simulink model "rectifire_single_inverter_pv1"  (R2022b)
settings: Solver=ode23tb  StartTime=0  StopTime=3  RelTol=1e-4
undefined symbols (not defined in the file): Ion, Lithium, P_100, sigbuilder_block, time_step
libraries: spsSeriesRLCBranchLib x26, spsTriangleGeneratorLib x26, slpidlib x26, spsVoltageMeasurementLib x14, spsCurrentMeasurementLib x11, spsDiodeLib x9, simulink x8, spsIGBTDiodeLib x8, spsMosfetLib x8, powerlib_extras x4, spsGroundLib x2, spsBatteryLib x2
(part 5 of 6)

== system rectifire_single_inverter_pv1/battery/Battery and DC-DC converter1/Modulation ==
  u1 : Inport
  u2 : Inport  Port=2
  NOT : Logic  Operator=NOT  AllPortsSameDT=off  OutDataTypeStr=boolean
  NOT1 : Logic  Operator=NOT  AllPortsSameDT=off  OutDataTypeStr=boolean
  Relational Operator : RelationalOperator  Operator=>  OutDataTypeStr=boolean  RndMeth=Simplest  InputSameDT=off
  Relational Operator1 : RelationalOperator  Operator=>  OutDataTypeStr=boolean  RndMeth=Simplest  InputSameDT=off
  Triangle Generator : spsTriangleGeneratorLib/Triangle Generator  Freq=wave_freq  Phase=0  Ts=0
  S1 : Outport
  S2 : Outport  Port=2
  S3 : Outport  Port=3
  S4 : Outport  Port=4
  wires:
  u1/1 -> Relational Operator/1
  Triangle Generator/1 -> Relational Operator1/2, Relational Operator/2
  u2/1 -> Relational Operator1/1
  Relational Operator/1 -> NOT/1, S1/1
  NOT/1 -> S2/1
  Relational Operator1/1 -> S4/1, NOT1/1
  NOT1/1 -> S3/1

== system rectifire_single_inverter_pv1/battery/Battery and DC-DC converter1/Modulation1 ==
  u1 : Inport
  u2 : Inport  Port=2
  NOT : Logic  Operator=NOT  AllPortsSameDT=off  OutDataTypeStr=boolean
  NOT1 : Logic  Operator=NOT  AllPortsSameDT=off  OutDataTypeStr=boolean
  Relational Operator : RelationalOperator  Operator=>  OutDataTypeStr=boolean  RndMeth=Simplest  InputSameDT=off
  Relational Operator1 : RelationalOperator  Operator=>  OutDataTypeStr=boolean  RndMeth=Simplest  InputSameDT=off
  Triangle Generator : spsTriangleGeneratorLib/Triangle Generator  Freq=wave_freq  Phase=0  Ts=0
  S1 : Outport
  S2 : Outport  Port=2
  S3 : Outport  Port=3
  S4 : Outport  Port=4
  wires:
  u1/1 -> Relational Operator/1
  Triangle Generator/1 -> Relational Operator1/2, Relational Operator/2
  u2/1 -> Relational Operator1/1
  Relational Operator/1 -> NOT/1, S1/1
  NOT/1 -> S2/1
  Relational Operator1/1 -> NOT1/1, S3/1
  NOT1/1 -> S4/1

== system rectifire_single_inverter_pv1/battery/Battery and DC-DC converter1/Modulation2 ==
  u1 : Inport
  u2 : Inport  Port=2
  NOT : Logic  Operator=NOT  AllPortsSameDT=off  OutDataTypeStr=boolean
  NOT1 : Logic  Operator=NOT  AllPortsSameDT=off  OutDataTypeStr=boolean
  Relational Operator : RelationalOperator  Operator=>  OutDataTypeStr=boolean  RndMeth=Simplest  InputSameDT=off
  Relational Operator1 : RelationalOperator  Operator=>  OutDataTypeStr=boolean  RndMeth=Simplest  InputSameDT=off
  Triangle Generator : spsTriangleGeneratorLib/Triangle Generator  Freq=wave_freq  Phase=0  Ts=0
  S1 : Outport
  S2 : Outport  Port=2
  S3 : Outport  Port=3
  S4 : Outport  Port=4
  wires:
  u1/1 -> Relational Operator/1
  Triangle Generator/1 -> Relational Operator1/2, Relational Operator/2
  u2/1 -> Relational Operator1/1
  Relational Operator/1 -> NOT/1, S1/1
  NOT/1 -> S2/1
  Relational Operator1/1 -> NOT1/1, S3/1
  NOT1/1 -> S4/1

== system rectifire_single_inverter_pv1/battery/Battery and DC-DC converter1/Modulation3 ==
  u1 : Inport
  u2 : Inport  Port=2
  NOT : Logic  Operator=NOT  AllPortsSameDT=off  OutDataTypeStr=boolean
  NOT1 : Logic  Operator=NOT  AllPortsSameDT=off  OutDataTypeStr=boolean
  Relational Operator : RelationalOperator  Operator=>  OutDataTypeStr=boolean  RndMeth=Simplest  InputSameDT=off
  Relational Operator1 : RelationalOperator  Operator=>  OutDataTypeStr=boolean  RndMeth=Simplest  InputSameDT=off
  Triangle Generator : spsTriangleGeneratorLib/Triangle Generator  Freq=wave_freq  Phase=0  Ts=0
  S1 : Outport
  S2 : Outport  Port=2
  S3 : Outport  Port=3
  S4 : Outport  Port=4
  wires:
  u1/1 -> Relational Operator/1
  Triangle Generator/1 -> Relational Operator1/2, Relational Operator/2
  u2/1 -> Relational Operator1/1
  Relational Operator/1 -> NOT/1, S1/1
  NOT/1 -> S2/1
  Relational Operator1/1 -> NOT1/1, S3/1
  NOT1/1 -> S4/1

== system rectifire_single_inverter_pv1/battery/Battery and DC-DC converter1/Modulation4 ==
  u1 : Inport
  u2 : Inport  Port=2
  NOT : Logic  Operator=NOT  AllPortsSameDT=off  OutDataTypeStr=boolean
  NOT1 : Logic  Operator=NOT  AllPortsSameDT=off  OutDataTypeStr=boolean
  Relational Operator : RelationalOperator  Operator=>  OutDataTypeStr=boolean  RndMeth=Simplest  InputSameDT=off
  Relational Operator1 : RelationalOperator  Operator=>  OutDataTypeStr=boolean  RndMeth=Simplest  InputSameDT=off
  Triangle Generator : spsTriangleGeneratorLib/Triangle Generator  Freq=wave_freq  Phase=0  Ts=0
  S1 : Outport
  S2 : Outport  Port=2
  S3 : Outport  Port=3
  S4 : Outport  Port=4
  wires:
  u1/1 -> Relational Operator/1
  Triangle Generator/1 -> Relational Operator1/2, Relational Operator/2
  u2/1 -> Relational Operator1/1
  Relational Operator/1 -> NOT/1, S1/1
  NOT/1 -> S2/1
  Relational Operator1/1 -> NOT1/1, S3/1
  NOT1/1 -> S4/1

== system rectifire_single_inverter_pv1/battery/Battery and DC-DC converter1/Modulation5 ==
  u1 : Inport
  u2 : Inport  Port=2
  NOT : Logic  Operator=NOT  AllPortsSameDT=off  OutDataTypeStr=boolean
  NOT1 : Logic  Operator=NOT  AllPortsSameDT=off  OutDataTypeStr=boolean
  Relational Operator : RelationalOperator  Operator=>  OutDataTypeStr=boolean  RndMeth=Simplest  InputSameDT=off
  Relational Operator1 : RelationalOperator  Operator=>  OutDataTypeStr=boolean  RndMeth=Simplest  InputSameDT=off
  Triangle Generator : spsTriangleGeneratorLib/Triangle Generator  Freq=wave_freq  Phase=0  Ts=0
  S1 : Outport
  S2 : Outport  Port=2
  S3 : Outport  Port=3
  S4 : Outport  Port=4
  wires:
  u1/1 -> Relational Operator/1
  Triangle Generator/1 -> Relational Operator1/2, Relational Operator/2
  u2/1 -> Relational Operator1/1
  Relational Operator/1 -> NOT/1, S1/1
  NOT/1 -> S2/1
  Relational Operator1/1 -> NOT1/1, S3/1
  NOT1/1 -> S4/1

== system rectifire_single_inverter_pv1/battery/Battery and DC-DC converter1/Modulation6 ==
  u1 : Inport
  u2 : Inport  Port=2
  NOT : Logic  Operator=NOT  AllPortsSameDT=off  OutDataTypeStr=boolean
  NOT1 : Logic  Operator=NOT  AllPortsSameDT=off  OutDataTypeStr=boolean
  Relational Operator : RelationalOperator  Operator=>  OutDataTypeStr=boolean  RndMeth=Simplest  InputSameDT=off
  Relational Operator1 : RelationalOperator  Operator=>  OutDataTypeStr=boolean  RndMeth=Simplest  InputSameDT=off
  Triangle Generator : spsTriangleGeneratorLib/Triangle Generator  Freq=wave_freq  Phase=0  Ts=0
  S1 : Outport
  S2 : Outport  Port=2
  S3 : Outport  Port=3
  S4 : Outport  Port=4
  wires:
  u1/1 -> Relational Operator/1
  Triangle Generator/1 -> Relational Operator1/2, Relational Operator/2
  u2/1 -> Relational Operator1/1
  Relational Operator/1 -> NOT/1, S1/1
  NOT/1 -> S2/1
  Relational Operator1/1 -> NOT1/1, S3/1
  NOT1/1 -> S4/1

== system rectifire_single_inverter_pv1/inverter/Subsystem/PWM1 ==
  In1 : Inport
  In2 : Inport  Port=2
  Constant : Constant
  Constant1 : Constant  Value=0
  Data Type Conversion1 : DataTypeConversion  OutDataTypeStr=boolean
  Subtract : Sum  Inputs=+-
  Switch : Switch  Threshold=0.5  SaturateOnIntegerOverflow=off  InputSameDT=off
  Out1 : Outport
  wires:
  Constant/1 -> Switch/1
  Subtract/1 -> Switch/2
  In2/1 -> Subtract/2
  In1/1 -> Subtract/1
  Switch/1 -> Data Type Conversion1/1
  Data Type Conversion1/1 -> Out1/1
  Constant1/1 -> Switch/3

== system rectifire_single_inverter_pv1/motor/SVPWM/PWM ==
  In : Inport
  Tcm123 : Inport  Port=2
  Add : Sum  Inputs=+-
  Add1 : Sum  Inputs=+-
  Add2 : Sum  Inputs=+-
  Data Type Conversion : DataTypeConversion  OutDataTypeStr=double  SaturateOnIntegerOverflow=off  RndMeth=Floor
  Data Type Conversion1 : DataTypeConversion  OutDataTypeStr=double  SaturateOnIntegerOverflow=off  RndMeth=Floor
  Data Type Conversion2 : DataTypeConversion  OutDataTypeStr=double  SaturateOnIntegerOverflow=off  RndMeth=Floor
  Demux : Demux  Outputs=3
  Logical Operator : Logic  Operator=NOT  AllPortsSameDT=off  OutDataTypeStr=boolean
  Logical Operator1 : Logic  Operator=NOT  AllPortsSameDT=off  OutDataTypeStr=boolean
  Logical Operator2 : Logic  Operator=NOT  AllPortsSameDT=off  OutDataTypeStr=boolean
  Mux : Mux  Inputs=6
  Relay : Relay  OffSwitchValue=-eps
  Relay1 : Relay  OffSwitchValue=-eps
  Relay2 : Relay  OffSwitchValue=-eps
  PWM : Outport  VectorParamsAs1DForOutWhenUnconnected=off
  wires:
  Demux/3 -> Add2/2
  Demux/2 -> Add1/2
  Demux/1 -> Add/2
  Relay2/1 -> Mux/5, Logical Operator2/1
  Relay1/1 -> Mux/3, Logical Operator1/1
  Relay/1 -> Logical Operator/1, Mux/1
  Mux/1 -> PWM/1
  Data Type Conversion/1 -> Mux/2
  Data Type Conversion1/1 -> Mux/4
  Data Type Conversion2/1 -> Mux/6
  Logical Operator2/1 -> Data Type Conversion2/1
  Logical Operator1/1 -> Data Type Conversion1/1
  Logical Operator/1 -> Data Type Conversion/1
  Add1/1 -> Relay1/1
  Add2/1 -> Relay2/1
  Add/1 -> Relay/1
  In/1 -> Add/1, Add2/1, Add1/1
  Tcm123/1 -> Demux/1

== system rectifire_single_inverter_pv1/motor/SVPWM/Sector Caculate ==
  Ualpha : Inport
  Ubeta : Inport  Port=2
  B0 : Fcn  Expr=u[2]
  B1 : Fcn  Expr=u[1]*sqrt(3/4)-0.5*u[2]
  B2 : Fcn  Expr=-u[1]*sqrt(3/4)-u[2]*0.5
  Constant : Constant
  Constant1 : Constant  Value=0
  Mux : Mux  Inputs=2
  Mux1 : Mux  Inputs=3
  N : Fcn  Expr=4*u[3]+2*u[2]+u[1]
  Switch : Switch  SaturateOnIntegerOverflow=off  InputSameDT=off
  Switch1 : Switch  SaturateOnIntegerOverflow=off  InputSameDT=off
  Switch2 : Switch  SaturateOnIntegerOverflow=off  InputSameDT=off
  "N " : Outport  VectorParamsAs1DForOutWhenUnconnected=off
  wires:
  Switch2/1 -> Mux1/3
  Switch/1 -> Mux1/1
  Ualpha/1 -> Mux/1
  Ubeta/1 -> Mux/2
  Mux/1 -> B2/1, B1/1, B0/1
  B0/1 -> Switch/2
  B1/1 -> Switch1/2
  B2/1 -> Switch2/2
  Constant/1 -> Switch/1, Switch2/1, Switch1/1
  Constant1/1 -> Switch/3, Switch1/3, Switch2/3
  Switch1/1 -> Mux1/2
  Mux1/1 -> N/1
  N/1 -> "N "/1

== system rectifire_single_inverter_pv1/motor/SVPWM/T1T1 Caculate ==
  note: T1
  note: T2
  N : Inport
  XYZ : Inport  Port=2
  Tpwm : Inport  Port=3
  Demux : Demux  Outputs=3
  Fcn : Fcn  Expr=u(3)-u(2)-u(1)
  Fcn1 : Fcn  Expr=u(1)*u(3)/(u(1)+u(2))
  Fcn2 : Fcn  Expr=u(2)*u(3)/(u(1)+u(2))
  Gain : Gain  Gain=-1
  Gain1 : Gain  Gain=-1
  Gain2 : Gain  Gain=-1
  Multiport Switch : MultiPortSwitch  Inputs=6  DiagnosticForDefault=None  SaturateOnIntegerOverflow=off  InputSameDT=off
  Multiport Switch1 : MultiPortSwitch  Inputs=6  DiagnosticForDefault=None  SaturateOnIntegerOverflow=off  InputSameDT=off
  Mux : Mux  Inputs=3
  Switch : Switch  SaturateOnIntegerOverflow=off  InputSameDT=off
  Switch1 : Switch  Criteria=u2 > Threshold  SaturateOnIntegerOverflow=off  InputSameDT=off
  T1 : Outport  VectorParamsAs1DForOutWhenUnconnected=off
  T2 : Outport  Port=2  VectorParamsAs1DForOutWhenUnconnected=off
  wires:
  Tpwm/1 -> Mux/3
  XYZ/1 -> Demux/1
  Switch1/1 -> T2/1
  Switch/1 -> T1/1
  Fcn2/1 -> Switch1/3
  Fcn1/1 -> Switch/3
  Fcn/1 -> Switch/2, Switch1/2
  Mux/1 -> Fcn1/1, Fcn/1, Fcn2/1
  Multiport Switch/1 -> Switch/1, Mux/1
  Multiport Switch1/1 -> Switch1/1, Mux/2
  N/1 -> Multiport Switch/1, Multiport Switch1/1
  Demux/2 -> Multiport Switch/3, Multiport Switch1/2, Gain1/1
  Demux/3 -> Multiport Switch1/5, Multiport Switch/2, Gain2/1
  Demux/1 -> Multiport Switch/6, Multiport Switch1/4, Gain/1
  Gain/1 -> Multiport Switch1/3, Multiport Switch/5
  Gain2/1 -> Multiport Switch/4, Multiport Switch1/7
  Gain1/1 -> Multiport Switch1/6, Multiport Switch/7

== system rectifire_single_inverter_pv1/motor/SVPWM/Tcm Caculate ==
  N : Inport
  T1 : Inport  Port=2
  T2 : Inport  Port=3
  Tpwm : Inport  Port=4
  Fcn : Fcn  Expr=(u[3]-u[1]-u[2])/4
  Fcn1 : Fcn  Expr=(u[3]+u[1]-u[2])/4
  Fcn2 : Fcn  Expr=(u[3]+u[2]+u[1])/4
  Multiport Switch : MultiPortSwitch  Inputs=6  DiagnosticForDefault=None  SaturateOnIntegerOverflow=off  InputSameDT=off
  Multiport Switch1 : MultiPortSwitch  Inputs=6  DiagnosticForDefault=None  SaturateOnIntegerOverflow=off  InputSameDT=off
  Multiport Switch2 : MultiPortSwitch  Inputs=6  DiagnosticForDefault=None  SaturateOnIntegerOverflow=off  InputSameDT=off
  Mux : Mux  Inputs=3
  Mux1 : Mux  Inputs=3
  Tcm1 Tcm2 Tcm3 : Outport  VectorParamsAs1DForOutWhenUnconnected=off
  wires:
  Mux/1 -> Fcn2/1, Fcn/1, Fcn1/1
  Tpwm/1 -> Mux/3
  T2/1 -> Mux/2
  T1/1 -> Mux/1
  Multiport Switch2/1 -> Mux1/3
  Multiport Switch1/1 -> Mux1/2
  Multiport Switch/1 -> Mux1/1
  Mux1/1 -> Tcm1 Tcm2 Tcm3/1
  Fcn/1 -> Multiport Switch/3, Multiport Switch/4, Multiport Switch1/6, Multiport Switch2/5, Multiport Switch2/7, Multiport Switch1/2
  Fcn1/1 -> Multiport Switch1/5, Multiport Switch2/3, Multiport Switch2/6, Multiport Switch1/4, Multiport Switch/7, Multiport Switch/2
  Fcn2/1 -> Multiport Switch/5, Multiport Switch/6, Multiport Switch1/3, Multiport Switch1/7, Multiport Switch2/2, Multiport Switch2/4
  N/1 -> Multiport Switch2/1, Multiport Switch1/1, Multiport Switch/1

== system rectifire_single_inverter_pv1/motor/SVPWM/XYZ Caculate ==
  Ualpha : Inport
  Ubeta : Inport  Port=2
  Ts : Inport  Port=3
  Udc : Inport  Port=4
  Add : Sum
  Add1 : Sum  Inputs=+-
  Gain : Gain  Gain=3/2
  Gain1 : Gain  Gain=sqrt(3)
  Gain2 : Gain  Gain=sqrt(3)/2
  Math Function : Math  Operator=reciprocal  SignedPower=on
  Mux : Mux  Inputs=3
  Product{,1..3} (4 alike) : Product  RndMeth=Zero
  XYZ : Outport  VectorParamsAs1DForOutWhenUnconnected=off
  wires:
  Mux/1 -> XYZ/1
  Product1/1 -> Mux/1
  Product3/1 -> Mux/2
  Product2/1 -> Mux/3
  Ualpha/1 -> Gain/1
  Ubeta/1 -> Gain2/1, Gain1/1
  Udc/1 -> Math Function/1
  Math Function/1 -> Product/2
  Ts/1 -> Product/1
  Gain1/1 -> Product1/1
  Product/1 -> Product2/2, Product1/2, Product3/2
  Gain/1 -> Add1/2, Add/2
  Gain2/1 -> Add/1, Add1/1
  Add1/1 -> Product2/1
  Add/1 -> Product3/1

== system rectifire_single_inverter_pv1/PV/PV module/PV module1/PV Current ==
  V : Inport
  T : Inport  Port=2
  I0 : Inport  Port=3
  Iph : Inport  Port=4
  Ish : Inport  Port=5
  Add1 : Sum
  Add2 : Sum  Inputs=+-
  Add3 : Sum  Inputs=+--
  Constant1 : Constant  Value=Rs
  Constant2 : Constant  Value=q
  Constant3 : Constant  Value=n
  Constant4 : Constant  Value=K
  Constant5 : Constant  Value=Ns
  Constant6 : Constant
  Math Function1 : Math
  Memory : Memory
  Product1 : Product
  Product2 : Product  Inputs=*////
  Product3 : Product
  Product4 : Product
  I : Outport
  wires:
  Add1/1 -> Product3/1
  V/1 -> Add1/1
  Add3/1 -> Memory/1, I/1
  Add2/1 -> Product4/2
  Product3/1 -> Math Function1/1
  Iph/1 -> Add3/1
  Product1/1 -> Add1/2
  Constant1/1 -> Product1/2
  Math Function1/1 -> Add2/1
  T/1 -> Product2/5
  Product2/1 -> Product3/2
  Constant5/1 -> Product2/4
  Constant3/1 -> Product2/2
  Constant4/1 -> Product2/3
  Constant2/1 -> Product2/1
  Product4/1 -> Add3/2
  I0/1 -> Product4/1
  Constant6/1 -> Add2/2
  Ish/1 -> Add3/3
  Memory/1 -> Product1/1

== system rectifire_single_inverter_pv1/PV/PV module/PV module1/Photo-current ==
  T : Inport
  G : Inport  Port=2
  Add1 : Sum  Inputs=+-
  Add2 : Sum
  Constant1 : Constant  Value=298
  Constant2 : Constant  Value=ki
  Constant3 : Constant  Value=Isc
  Constant4 : Constant  Value=1000
  Product1 : Product
  Product2 : Product
  Product3 : Product  Inputs=*/
  Iph : Outport
  wires:
  T/1 -> Add1/1
  G/1 -> Product2/1
  Product1/1 -> Add2/2
  Constant4/1 -> Product3/2
  Constant2/1 -> Product1/2
  Product3/1 -> Iph/1
  Constant3/1 -> Add2/1
  Add1/1 -> Product1/1
  Constant1/1 -> Add1/2
  Add2/1 -> Product2/2
  Product2/1 -> Product3/1

== system rectifire_single_inverter_pv1/PV/PV module/PV module1/Reverse Saturation Current ==
  T : Inport
  Add : Sum  Inputs=+-
  Constant2 : Constant  Value=q  SampleTime=-1
  Constant3 : Constant  Value=Voc  SampleTime=-1
  Constant4 : Constant  Value=n  SampleTime=-1
  Constant5 : Constant  VectorParams1D=off  SampleTime=-1
  Constant6 : Constant  Value=K  SampleTime=-1
  Constant7 : Constant  Value=Ns  SampleTime=-1
  Constant8 : Constant  Value=Isc  SampleTime=-1
  Math Function1 : Math
  Product1 : Product
  Product2 : Product  Inputs=4
  Product3 : Product  Inputs=*/
  Product4 : Product  Inputs=*/
  Irc : Outport
  wires:
  Product4/1 -> Irc/1
  Product2/1 -> Product3/2
  T/1 -> Product2/4
  Constant5/1 -> Add/2
  Constant2/1 -> Product1/1
  Product3/1 -> Math Function1/1
  Add/1 -> Product4/2
  Constant8/1 -> Product4/1
  Constant3/1 -> Product1/2
  Constant7/1 -> Product2/2
  Constant4/1 -> Product2/1
  Constant6/1 -> Product2/3
  Math Function1/1 -> Add/1
  Product1/1 -> Product3/1

== system rectifire_single_inverter_pv1/PV/PV module/PV module1/Saturation current ==
  T : Inport
  Irs : Inport  Port=2
  Add : Sum  Inputs=+-
  Constant10 : Constant  Value=3  VectorParams1D=off  SampleTime=-1
  Constant2 : Constant  VectorParams1D=off  SampleTime=-1
  Constant3 : Constant  Value=Tn  SampleTime=-1
  Constant4 : Constant  VectorParams1D=off  SampleTime=-1
  Constant5 : Constant  Value=q  SampleTime=-1
  Constant6 : Constant  Value=Eg0  SampleTime=-1
  Constant7 : Constant  Value=n  SampleTime=-1
  Constant8 : Constant  Value=K  SampleTime=-1
  Constant9 : Constant  Value=Tn  SampleTime=-1
  Math Function1 : Math
  Math Function2 : Math  Operator=pow
  Product{1..2,5..6} (4 alike) : Product  Inputs=*/
  Product3 : Product  Inputs=3
  Product4 : Product
  Product7 : Product  Inputs=3
  I0 : Outport
  wires:
  T/1 -> Product2/2, Product6/1
  Constant7/1 -> Product4/1
  Product6/1 -> Math Function2/1
  Math Function1/1 -> Product7/3
  Constant2/1 -> Product1/1
  Constant4/1 -> Product2/1
  Product3/1 -> Product5/1
  Add/1 -> Product3/3
  Irs/1 -> Product7/1
  Constant3/1 -> Product1/2
  Math Function2/1 -> Product7/2
  Constant10/1 -> Math Function2/2
  Product1/1 -> Add/1
  Constant8/1 -> Product4/2
  Constant9/1 -> Product6/2
  Product4/1 -> Product5/2
  Constant6/1 -> Product3/2
  Product7/1 -> I0/1
  Product5/1 -> Math Function1/1
  Constant5/1 -> Product3/1
  Product2/1 -> Add/2

== system rectifire_single_inverter_pv1/PV/PV module/PV module1/Shunt Current ==
  I : Inport
  V : Inport  Port=2
  Add : Sum
  Constant1 : Constant  Value=Rs  SampleTime=-1
  Constant2 : Constant  Value=Rsh  SampleTime=-1
  Product1 : Product
  Product2 : Product  Inputs=*/
  Ish : Outport
  wires:
  I/1 -> Product1/1
  Constant1/1 -> Product1/2
  Product2/1 -> Ish/1
  Constant2/1 -> Product2/2
  V/1 -> Add/2
  Add/1 -> Product2/1
  Product1/1 -> Add/1

== system rectifire_single_inverter_pv1/battery/Battery and DC-DC converter/Charge Mixed CurrentPower/Modulation ==
  u1 : Inport
  u2 : Inport  Port=2
  triangular_generator : Inport  Port=3
  NOT : Logic  Operator=NOT  AllPortsSameDT=off  OutDataTypeStr=boolean
  NOT1 : Logic  Operator=NOT  AllPortsSameDT=off  OutDataTypeStr=boolean
  Relational Operator : RelationalOperator  Operator=>  OutDataTypeStr=boolean  RndMeth=Simplest  InputSameDT=off
  Relational Operator1 : RelationalOperator  Operator=>  OutDataTypeStr=boolean  RndMeth=Simplest  InputSameDT=off
  Triangle Generator : spsTriangleGeneratorLib/Triangle Generator  Commented=on  Freq=wave_freq  Phase=0  Ts=0
  S1 : Outport
  S2 : Outport  Port=2
  S3 : Outport  Port=3
  S4 : Outport  Port=4
  wires:
  u1/1 -> Relational Operator/1
  triangular_generator/1 -> Relational Operator1/2, Relational Operator/2
  u2/1 -> Relational Operator1/1
  NOT1/1 -> S4/1
  Relational Operator/1 -> S1/1, NOT/1
  Relational Operator1/1 -> S3/1, NOT1/1
  NOT/1 -> S2/1

== system rectifire_single_inverter_pv1/battery/Battery and DC-DC converter/Charge Mixed CurrentPower1/Modulation ==
  u1 : Inport
  u2 : Inport  Port=2
  triangular_generator : Inport  Port=3
  NOT : Logic  Operator=NOT  AllPortsSameDT=off  OutDataTypeStr=boolean
  NOT1 : Logic  Operator=NOT  AllPortsSameDT=off  OutDataTypeStr=boolean
  Relational Operator : RelationalOperator  Operator=>  OutDataTypeStr=boolean  RndMeth=Simplest  InputSameDT=off
  Relational Operator1 : RelationalOperator  Operator=>  OutDataTypeStr=boolean  RndMeth=Simplest  InputSameDT=off
  Triangle Generator : spsTriangleGeneratorLib/Triangle Generator  Commented=on  Freq=wave_freq  Phase=0  Ts=0
  S1 : Outport
  S2 : Outport  Port=2
  S3 : Outport  Port=3
  S4 : Outport  Port=4
  wires:
  u1/1 -> Relational Operator/1
  triangular_generator/1 -> Relational Operator1/2, Relational Operator/2
  u2/1 -> Relational Operator1/1
  NOT1/1 -> S4/1
  Relational Operator/1 -> S1/1, NOT/1
  Relational Operator1/1 -> S3/1, NOT1/1
  NOT/1 -> S2/1

== system rectifire_single_inverter_pv1/battery/Battery and DC-DC converter/Discharge Const Voltage/Modulation ==
  u1 : Inport
  u2 : Inport  Port=2
  triangular_generator : Inport  Port=3
  NOT : Logic  Operator=NOT  AllPortsSameDT=off  OutDataTypeStr=boolean
  NOT1 : Logic  Operator=NOT  AllPortsSameDT=off  OutDataTypeStr=boolean
  Relational Operator : RelationalOperator  Operator=>  OutDataTypeStr=boolean  RndMeth=Simplest  InputSameDT=off
  Relational Operator1 : RelationalOperator  Operator=>  OutDataTypeStr=boolean  RndMeth=Simplest  InputSameDT=off
  Triangle Generator : spsTriangleGeneratorLib/Triangle Generator  Commented=on  Freq=wave_freq  Phase=0  Ts=0
  S1 : Outport
  S2 : Outport  Port=2
  S3 : Outport  Port=3
  S4 : Outport  Port=4
  wires:
  u1/1 -> Relational Operator/1
  triangular_generator/1 -> Relational Operator1/2, Relational Operator/2
  u2/1 -> Relational Operator1/1
  NOT1/1 -> S4/1
  Relational Operator/1 -> S1/1, NOT/1
  Relational Operator1/1 -> S3/1, NOT1/1
  NOT/1 -> S2/1

== system rectifire_single_inverter_pv1/battery/Battery and DC-DC converter/Discharge Mixed CurrentPower/Modulation ==
  u1 : Inport
  u2 : Inport  Port=2
  triangular_generator : Inport  Port=3
  NOT : Logic  Operator=NOT  AllPortsSameDT=off  OutDataTypeStr=boolean
  NOT1 : Logic  Operator=NOT  AllPortsSameDT=off  OutDataTypeStr=boolean
  Relational Operator : RelationalOperator  Operator=>  OutDataTypeStr=boolean  RndMeth=Simplest  InputSameDT=off
  Relational Operator1 : RelationalOperator  Operator=>  OutDataTypeStr=boolean  RndMeth=Simplest  InputSameDT=off
  Triangle Generator : spsTriangleGeneratorLib/Triangle Generator  Commented=on  Freq=wave_freq  Phase=0  Ts=0
  S1 : Outport
  S2 : Outport  Port=2
  S3 : Outport  Port=3
  S4 : Outport  Port=4
  wires:
  u1/1 -> Relational Operator/1
  triangular_generator/1 -> Relational Operator1/2, Relational Operator/2
  u2/1 -> Relational Operator1/1
  NOT1/1 -> S4/1
  Relational Operator/1 -> S1/1, NOT/1
  Relational Operator1/1 -> S3/1, NOT1/1
  NOT/1 -> S2/1

== system rectifire_single_inverter_pv1/battery/Battery and DC-DC converter1/Charge Mixed CurrentPower1/Modulation ==
  u1 : Inport
  u2 : Inport  Port=2
  triangular_generator : Inport  Port=3
  NOT : Logic  Operator=NOT  AllPortsSameDT=off  OutDataTypeStr=boolean
  NOT1 : Logic  Operator=NOT  AllPortsSameDT=off  OutDataTypeStr=boolean
  Relational Operator : RelationalOperator  Operator=>  OutDataTypeStr=boolean  RndMeth=Simplest  InputSameDT=off
  Relational Operator1 : RelationalOperator  Operator=>  OutDataTypeStr=boolean  RndMeth=Simplest  InputSameDT=off
  Triangle Generator : spsTriangleGeneratorLib/Triangle Generator  Commented=on  Freq=wave_freq  Phase=0  Ts=0
  S1 : Outport
  S2 : Outport  Port=2
  S3 : Outport  Port=3
  S4 : Outport  Port=4
  wires:
  u1/1 -> Relational Operator/1
  triangular_generator/1 -> Relational Operator1/2, Relational Operator/2
  u2/1 -> Relational Operator1/1
  NOT1/1 -> S4/1
  Relational Operator/1 -> S1/1, NOT/1
  Relational Operator1/1 -> S3/1, NOT1/1
  NOT/1 -> S2/1

== system rectifire_single_inverter_pv1/battery/Battery and DC-DC converter1/Discharge Const Voltage/Modulation ==
  u1 : Inport
  u2 : Inport  Port=2
  triangular_generator : Inport  Port=3
  NOT : Logic  Operator=NOT  AllPortsSameDT=off  OutDataTypeStr=boolean
  NOT1 : Logic  Operator=NOT  AllPortsSameDT=off  OutDataTypeStr=boolean
  Relational Operator : RelationalOperator  Operator=>  OutDataTypeStr=boolean  RndMeth=Simplest  InputSameDT=off
  Relational Operator1 : RelationalOperator  Operator=>  OutDataTypeStr=boolean  RndMeth=Simplest  InputSameDT=off
  Triangle Generator : spsTriangleGeneratorLib/Triangle Generator  Commented=on  Freq=wave_freq  Phase=0  Ts=0
  S1 : Outport
  S2 : Outport  Port=2
  S3 : Outport  Port=3
  S4 : Outport  Port=4
  wires:
  u1/1 -> Relational Operator/1
  triangular_generator/1 -> Relational Operator1/2, Relational Operator/2
  u2/1 -> Relational Operator1/1
  NOT1/1 -> S3/1
  Relational Operator/1 -> S1/1, NOT/1
  Relational Operator1/1 -> S4/1, NOT1/1
  NOT/1 -> S2/1

== matlab function rectifire_single_inverter_pv1/battery/Battery and DC-DC converter1/MATLAB Function4 ==
  data: discharge_mode_flag input; v_battery input; block_status output; v_bus input; i_battery input; i_bus input
function block_status = CurrentVoltageProtection(discharge_mode_flag, v_battery, v_bus, i_battery, i_bus)
% Input Voltage / Output current Protection Module
% param discharge_mode_flag: direction,
%    0-charge the inner battery; 1-battery discharge
%% Protection Voltage/Current Value
input_lack_voltage_point_bus = 85.0;
input_lack_voltage_recover_point_bus = 87.0;
input_lack_voltage_point_battery = 80.0;
input_lack_voltage_recover_point_battery = 83.0;

input_over_voltage_point_bus = 122;
input_over_voltage_recover_point_bus = 120;
input_over_voltage_point_battery = 120;
input_over_voltage_recover_point_battery = 118;

output_over_current_point_bus = 32;  % discharge
output_over_current_point_battery = 33; % charge


block_flag = true;
discharge_flag = true;

persistent current_block_status;
if isempty(current_block_status)
    current_block_status = ~block_flag;
end
block_status = current_block_status;

%% charge the battery
if (discharge_mode_flag == ~discharge_flag && current_block_status == ~block_flag)

    if (v_bus < input_lack_voltage_point_bus) || (v_bus > input_over_voltage_point_bus) || ...
            (i_battery > output_over_current_point_battery)
        block_status = block_flag;
    else 
        block_status = ~block_flag;
    end

end


if (discharge_mode_flag == ~discharge_flag && current_block_status == block_flag)
    % has been blocked in charging
    if (v_bus > input_lack_voltage_recover_point_bus) && (v_bus < input_over_voltage_recover_point_bus) && ...
        (i_battery < output_over_current_point_battery)
        block_status = ~block_flag;
    else
        block_status = block_flag;
    end
end

%% disharge the battery
if (discharge_mode_flag == discharge_flag && current_block_status == ~block_flag)

    if (v_battery < input_lack_voltage_point_battery) || (v_battery > input_over_voltage_point_battery) || ...
            (i_bus > output_over_current_point_battery)
        block_status = block_flag;
    else 
        block_status = ~block_flag;
    end

end


if (discharge_mode_flag == discharge_flag && current_block_status == block_flag)
    % has been blocked
    if (v_battery > input_lack_voltage_recover_point_battery) && (v_battery < input_over_voltage_recover_point_battery) && ...
            (i_bus < output_over_current_point_battery)
        block_status = ~block_flag;
    else
        block_status = block_flag;
    end
end

current_block_status = block_status;

== matlab function rectifire_single_inverter_pv1/battery/Battery and DC-DC converter1/MATLAB Function6 ==
  settings: updateMethod=DISCRETE
  data: iL_ref input; u1 output; iL input; i_out_ref input; i_out input; vin input; Vc input; Ts input; u2 output
function [u1, u2] = Passivity_BC(iL_ref, iL,i_out_ref, i_out, vin, Vc, Ts)
% Constant output current Module
% param iL: inductor's current
% param iL_ref: expected value of inductor's current
% param i_out: dcdc output current 
% param i_out_ref
% param vin: input voltage
% param Vc: output voltage
%% system parameters
L = 40e-6;  % Inductance 电感 20uH
L_DMinductor = 2.2e-6;
L = L + L_DMinductor;
RL = 0.004;
C_output = 1440e-6;  % 电容大小

zeta1 = 6;  % dumping gains
zeta2 = 0.08;

% error functions: state variable
x1 = iL - iL_ref;
x2 = i_out - i_out_ref;
persistent iL_ref_old Vc_old;
if isempty(iL_ref_old)
    iL_ref_old = 0;
    Vc_old = 0;
end

diL_ref = (iL_ref - iL_ref_old) / Ts;
dVc_ref = (Vc - Vc_old) / Ts;
%% calculate switching signal: u1,u2
u2 = 1 / iL_ref * (iL_ref - C_output * dVc_ref - i_out_ref + x2*zeta2);
u1 = 1 / vin * (L*diL_ref + RL * iL_ref + Vc * (1 - u2) - x1*zeta1);

iL_ref_old = iL_ref;
Vc_old = Vc;

== matlab function rectifire_single_inverter_pv1/battery/Battery and DC-DC converter1/MATLAB Function7 ==
  settings: updateMethod=DISCRETE
  data: iL_ref input; u1 output; iL input; vc_ref input; vc input; vin input; i_out input; Ts input; u2 output; Bus_load input
function [u1, u2] = Passivity_BC(iL_ref, iL, vc_ref, vc, vin, i_out, Ts, Bus_load)
% Constant output voltage Module
%   param vc_ref: expected
%   param vc: dcdc output voltage
%   param vin: input voltage
%   param io: current in output side
%   param Bus_load:
%% system parameters
L = 40e-6;  % Inductance 电感 20uH
L_DMinductor = 2.2e-6;
L = L + L_DMinductor;
RL = 0.004;
Co = 1440e-6;  % 电容大小

zeta1 = L / RL * 2000;  % dumping gains
zeta2 = Co * 1000; 

% if Bus_load > 1e4
%     zeta2 = 1e-3;
% end


% error functions: state variable
x1 = iL - iL_ref;
x2 = vc - vc_ref;
persistent iL_ref_old vc_ref_old;
if isempty(iL_ref_old)
    iL_ref_old = 0;
    vc_ref_old = 0;
end

diL_ref = (iL_ref - iL_ref_old) / Ts;
dvc_ref = (vc_ref - vc_ref_old) / Ts;
%% calculate switching signal: u1,u2
% u2 denotes S3's state
% u1 denotes S1's state
u2 = 1 / iL_ref * (iL_ref - dvc_ref * Co - i_out + x2*zeta2);
u1 = 1 / vin * (L*diL_ref + RL*iL_ref + vc_ref*(1-u2) - x1*zeta1);
iL_ref_old = iL_ref;
vc_ref_old = vc_ref;

% compensate strategy
S1_duty_cycle = vc_ref / vin;
S4_duty_cycle = 1 - vin / vc_ref;  % vin < vc
S3_duty_cycle = 1- S4_duty_cycle;
PWM_triangular_wave_range = 2;
PWM_triangular_wave_min = -1;
original_u2 = u2;


persistent voltage_surge_max;
if isempty(voltage_surge_max)
    voltage_surge_max = 0;
end

if Bus_load > 1e2
    u2 = S4_duty_cycle;  % need to check
end

% if Bus_load > 1e2 && abs(vc - vc_ref) < 0.2
%     u2 = 0.5 * PWM_triangular_wave_range + PWM_triangular_wave_min;
%     u1 = 0.5 * PWM_triangular_wave_range + PWM_triangular_wave_min;
% end

if vc - vc_ref > 1 && (vc - voltage_surge_max > -0.4)
%     u2 = 2;
    u2 = S3_duty_cycle * PWM_triangular_wave_range + PWM_triangular_wave_min;
end
if vc - vc_ref > 1 && vin - vc_ref > 1
    u1 = (1 - S1_duty_cycle) * PWM_triangular_wave_range + PWM_triangular_wave_min;
end

% solve buck-boost mode: sudden u2=1, keep bucking
if vc_ref -vc > 0.2 && Bus_load > 1e2
    % In buck-boost mode, start boost when vc starts to drop > 0.3V
    u2 = S4_duty_cycle;
    u1 = max(u1, S3_duty_cycle* PWM_triangular_wave_range + PWM_triangular_wave_min);
end

% % Boost mode
% if (vc_ref - vin) > 1 && (vc_ref - vc) > 0.5
%     u1 = S1_duty_cycle * PWM_triangular_wave_range + PWM_triangular_wave_min;
% %     u2 = S4_duty_cycle * PWM_triangular_wave_range + PWM_triangular_wave_min;
% end
% 
% % Buck mode
% if vin - vc_ref > 1 && vc - vc_ref > 1
%     u2 = 2;
% %     u1 = S1_duty_cycle * PWM_triangular_wave_range + PWM_triangular_wave_min;
% end

voltage_surge_max = max(vc, voltage_surge_max);

== matlab function rectifire_single_inverter_pv1/battery/Battery and DC-DC converter1/Charge Mixed CurrentPower1/MATLAB Function3 ==
  settings: updateMethod=DISCRETE
  data: iL_ref input; u1 output; iL input; i_out_ref input; i_out input; vin input; Vc input; Ts input; u2 output
function [u1, u2] = Passivity_BC(iL_ref, iL,i_out_ref, i_out, vin, Vc, Ts)
% Constant output current Module
% param iL: inductor's current
% param iL_ref: expected value of inductor's current
% param i_out: dcdc output current 
% param i_out_ref
% param vin: input voltage
% param Vc: output voltage
%% system parameters
L = 40e-6;  % Inductance 电感 20uH
L_DMinductor = 2.2e-6;
L = L + L_DMinductor;
RL = 0.004;
C_output = 1440e-6;  % 电容大小

% zeta1 = 6 * 2;  % dumping gains
% zeta2 = 0.08 * 10;
zeta1 = L / RL * 2000;  % dumping gains
zeta2 = C_output * 1000; 

% error functions: state variable
x1 = iL - iL_ref;
x2 = i_out - i_out_ref;
persistent iL_ref_old Vc_old;
if isempty(iL_ref_old)
    iL_ref_old = 0;
    Vc_old = 0;
end

diL_ref = (iL_ref - iL_ref_old) / Ts;
dVc_ref = (Vc - Vc_old) / Ts;
%% calculate switching signal: u1,u2
u2 = 1 / iL_ref * (iL_ref - C_output * dVc_ref - i_out_ref + x2*zeta2);
u1 = 1 / vin * (L*diL_ref + RL * iL_ref + Vc * (1 - u2) - x1*zeta1);

iL_ref_old = iL_ref;
Vc_old = Vc;

== matlab function rectifire_single_inverter_pv1/battery/Battery and DC-DC converter/Charge Mixed CurrentPower/MATLAB Function1 ==
  settings: updateMethod=DISCRETE
  data: iL_ref input; u1 output; iL input; i_out_ref input; i_out input; vin input; Vc input; Ts input; u2 output
function [u1, u2] = Passivity_BC(iL_ref, iL,i_out_ref, i_out, vin, Vc, Ts)
% Constant output current Module
% param iL: inductor's current
% param iL_ref: expected value of inductor's current
% param i_out: dcdc output current 
% param i_out_ref
% param vin: input voltage
% param Vc: output voltage
%% system parameters
L = 40e-6;  % Inductance 电感 20uH
L_DMinductor = 2.2e-6;
L = L + L_DMinductor;
RL = 0.004;
C_output = 1440e-6;  % 电容大小

zeta1 = 6;  % dumping gains
zeta2 = 0.08;

% error functions: state variable
x1 = iL - iL_ref;
x2 = i_out - i_out_ref;
persistent iL_ref_old Vc_old;
if isempty(iL_ref_old)
    iL_ref_old = 0;
    Vc_old = 0;
end

diL_ref = (iL_ref - iL_ref_old) / Ts;
dVc_ref = (Vc - Vc_old) / Ts;
%% calculate switching signal: u1,u2
u2 = 1 / iL_ref * (iL_ref - C_output * dVc_ref - i_out_ref + x2*zeta2);
u1 = 1 / vin * (L*diL_ref + RL * iL_ref + Vc * (1 - u2) - x1*zeta1);

iL_ref_old = iL_ref;
Vc_old = Vc;

== matlab function rectifire_single_inverter_pv1/battery/Battery and DC-DC converter1/MATLAB Function1 ==
  settings: updateMethod=DISCRETE
  data: iL_ref input; u1 output; iL input; i_out_ref input; i_out input; vin input; Vc input; Ts input; u2 output
function [u1, u2] = Passivity_BC(iL_ref, iL,i_out_ref, i_out, vin, Vc, Ts)
% Constant output current Module
% param iL: inductor's current
% param iL_ref: expected value of inductor's current
% param i_out: dcdc output current 
% param i_out_ref
% param vin: input voltage
% param Vc: output voltage
%% system parameters
L = 40e-6;  % Inductance 电感 20uH
L_DMinductor = 2.2e-6;
L = L + L_DMinductor;
RL = 0.004;
C_output = 1440e-6;  % 电容大小

% zeta1 = 6*2;  % dumping gains
% zeta2 = 0.08*10;
zeta1 = L / RL * 2000;  % dumping gains
zeta2 = C_output * 1000; 

% error functions: state variable
x1 = iL - iL_ref;
x2 = i_out - i_out_ref;
persistent iL_ref_old Vc_old;
if isempty(iL_ref_old)
    iL_ref_old = 0;
    Vc_old = 0;
end

diL_ref = (iL_ref - iL_ref_old) / Ts;
dVc_ref = (Vc - Vc_old) / Ts;
%% calculate switching signal: u1,u2
u2 = 1 / iL_ref * (iL_ref - C_output * dVc_ref - i_out_ref + x2*zeta2);
u1 = 1 / vin * (L*diL_ref + RL * iL_ref + Vc * (1 - u2) - x1*zeta1);

iL_ref_old = iL_ref;
Vc_old = Vc;

== matlab function rectifire_single_inverter_pv1/battery/Battery and DC-DC converter/Charge Mixed CurrentPower1/MATLAB Function3 ==
  settings: updateMethod=DISCRETE
  data: iL_ref input; u1 output; iL input; i_out_ref input; i_out input; vin input; Vc input; Ts input; u2 output
function [u1, u2] = Passivity_BC(iL_ref, iL,i_out_ref, i_out, vin, Vc, Ts)
% Constant output current Module
% param iL: inductor's current
% param iL_ref: expected value of inductor's current
% param i_out: dcdc output current 
% param i_out_ref
% param vin: input voltage
% param Vc: output voltage
%% system parameters
L = 40e-6;  % Inductance 电感 20uH
L_DMinductor = 2.2e-6;
L = L + L_DMinductor;
RL = 0.004;
C_output = 1440e-6;  % 电容大小

% zeta1 = 6 * 2;  % dumping gains
% zeta2 = 0.08 * 10;
zeta1 = L / RL * 2000;  % dumping gains
zeta2 = C_output * 1000; 

% error functions: state variable
x1 = iL - iL_ref;
x2 = i_out - i_out_ref;
persistent iL_ref_old Vc_old;
if isempty(iL_ref_old)
    iL_ref_old = 0;
    Vc_old = 0;
end

diL_ref = (iL_ref - iL_ref_old) / Ts;
dVc_ref = (Vc - Vc_old) / Ts;
%% calculate switching signal: u1,u2
u2 = 1 / iL_ref * (iL_ref - C_output * dVc_ref - i_out_ref + x2*zeta2);
u1 = 1 / vin * (L*diL_ref + RL * iL_ref + Vc * (1 - u2) - x1*zeta1);

iL_ref_old = iL_ref;
Vc_old = Vc;

== matlab function rectifire_single_inverter_pv1/battery/Battery and DC-DC converter/Discharge Const Voltage/MATLAB Function1 ==
  settings: updateMethod=DISCRETE
  data: iL_ref input; u1 output; iL input; vc_ref input; vc input; vin input; i_out input; Ts input; u2 output; Bus_load input
function [u1, u2] = Passivity_BC(iL_ref, iL, vc_ref, vc, vin, i_out, Ts, Bus_load)
% Constant output voltage Module
%   param vc_ref: expected
%   param vc: dcdc output voltage
%   param vin: input voltage
%   param io: current in output side
%   param Bus_load:
%% system parameters
L = 40e-6;  % Inductance 电感 20uH
L_DMinductor = 2.2e-6;
L = L + L_DMinductor;
RL = 0.004;
Co = 1440e-6;  % 电容大小

zeta1 = L / RL * 2000;  % dumping gains
zeta2 = Co * 1000; 

% if Bus_load > 1e4
%     zeta2 = 1e-3;
% end


% error functions: state variable
x1 = iL - iL_ref;
x2 = vc - vc_ref;
persistent iL_ref_old vc_ref_old;
if isempty(iL_ref_old)
    iL_ref_old = 0;
    vc_ref_old = 0;
end

diL_ref = (iL_ref - iL_ref_old) / Ts;
dvc_ref = (vc_ref - vc_ref_old) / Ts;
%% calculate switching signal: u1,u2
% u2 denotes S3's state
% u1 denotes S1's state
u2 = 1 / iL_ref * (iL_ref - dvc_ref * Co - i_out + x2*zeta2);
u1 = 1 / vin * (L*diL_ref + RL*iL_ref + vc_ref*(1-u2) - x1*zeta1);
iL_ref_old = iL_ref;
vc_ref_old = vc_ref;

% compensate strategy
S1_duty_cycle = vc_ref / vin;
S4_duty_cycle = 1 - vin / vc_ref;  % vin < vc
S3_duty_cycle = 1- S4_duty_cycle;
PWM_triangular_wave_range = 2;
PWM_triangular_wave_min = -1;
original_u2 = u2;


persistent voltage_surge_max;
if isempty(voltage_surge_max)
    voltage_surge_max = 0;
end

if Bus_load > 1e2
    u2 = S4_duty_cycle;  % need to check
end

% if Bus_load > 1e2 && abs(vc - vc_ref) < 0.2
%     u2 = 0.5 * PWM_triangular_wave_range + PWM_triangular_wave_min;
%     u1 = 0.5 * PWM_triangular_wave_range + PWM_triangular_wave_min;
% end

if vc - vc_ref > 1 % && (vc - voltage_surge_max > -0.4)
%     u2 = 2;
    u2 = S3_duty_cycle * PWM_triangular_wave_range + PWM_triangular_wave_min;
end
if vc - vc_ref > 1 && vin - vc_ref > 1
    u1 = (1 - S1_duty_cycle) * PWM_triangular_wave_range + PWM_triangular_wave_min;
end

% solve buck-boost mode: sudden u2=1, keep bucking
if vc_ref -vc > 0.2 && Bus_load > 1e2
    % In buck-boost mode, start boost when vc starts to drop > 0.3V
    u2 = S4_duty_cycle;
    u1 = max(u1, S3_duty_cycle* PWM_triangular_wave_range + PWM_triangular_wave_min);
end

% % Boost mode
% if (vc_ref - vin) > 1 && (vc_ref - vc) > 0.5
%     u1 = S1_duty_cycle * PWM_triangular_wave_range + PWM_triangular_wave_min;
% %     u2 = S4_duty_cycle * PWM_triangular_wave_range + PWM_triangular_wave_min;
% end
% 
% % Buck mode
% if vin - vc_ref > 1 && vc - vc_ref > 1
%     u2 = 2;
% %     u1 = S1_duty_cycle * PWM_triangular_wave_range + PWM_triangular_wave_min;
% end

voltage_surge_max = max(vc, voltage_surge_max);

== matlab function rectifire_single_inverter_pv1/battery/Battery and DC-DC converter/Discharge Mixed CurrentPower/MATLAB Function2 ==
  settings: updateMethod=DISCRETE
  data: iL_ref input; u1 output; iL input; i_out_ref input; i_out input; vin input; Vc input; Ts input; u2 output
function [u1, u2] = Passivity_BC(iL_ref, iL,i_out_ref, i_out, vin, Vc, Ts)
% Constant output current Module
% param iL: inductor's current
% param iL_ref: expected value of inductor's current
% param i_out: dcdc output current 
% param i_out_ref
% param vin: input voltage
% param Vc: output voltage
%% system parameters
L = 40e-6;  % Inductance 电感 20uH
L_DMinductor = 2.2e-6;
L = L + L_DMinductor;
RL = 0.004;
C_output = 1440e-6;  % 电容大小

zeta1 = 6*2;  % dumping gains
zeta2 = 0.08*10;

% error functions: state variable
x1 = iL - iL_ref;
x2 = i_out - i_out_ref;
persistent iL_ref_old Vc_old;
if isempty(iL_ref_old)
    iL_ref_old = 0;
    Vc_old = 0;
end

diL_ref = (iL_ref - iL_ref_old) / Ts;
dVc_ref = (Vc - Vc_old) / Ts;
%% calculate switching signal: u1,u2
u2 = 1 / iL_ref * (iL_ref - C_output * dVc_ref - i_out_ref + x2*zeta2);
u1 = 1 / vin * (L*diL_ref + RL * iL_ref + Vc * (1 - u2) - x1*zeta1);

iL_ref_old = iL_ref;
Vc_old = Vc;

== matlab function rectifire_single_inverter_pv1/battery/Battery and DC-DC converter/MATLAB Function ==
  settings: updateMethod=DISCRETE
  data: iL_ref input; u1 output; iL input; vc_ref input; vc input; vin input; i_out input; Ts input; u2 output; Bus_load input
function [u1, u2] = Passivity_BC(iL_ref, iL, vc_ref, vc, vin, i_out, Ts, Bus_load)
% Constant output voltage Module
%   param vc_ref: expected
%   param vc: dcdc output voltage
%   param vin: input voltage
%   param io: current in output side
%   param Bus_load:
%% system parameters
L = 40e-6;  % Inductance 电感 20uH
L_DMinductor = 2.2e-6;
L = L + L_DMinductor;
RL = 0.004;
Co = 1440e-6;  % 电容大小

zeta1 = L / RL * 2000;  % dumping gains
zeta2 = Co * 1000; 

% if Bus_load > 1e4
%     zeta2 = 1e-3;
% end


% error functions: state variable
x1 = iL - iL_ref;
x2 = vc - vc_ref;
persistent iL_ref_old vc_ref_old;
if isempty(iL_ref_old)
    iL_ref_old = 0;
    vc_ref_old = 0;
end

diL_ref = (iL_ref - iL_ref_old) / Ts;
dvc_ref = (vc_ref - vc_ref_old) / Ts;
%% calculate switching signal: u1,u2
% u2 denotes S3's state
% u1 denotes S1's state
u2 = 1 / iL_ref * (iL_ref - dvc_ref * Co - i_out + x2*zeta2);
u1 = 1 / vin * (L*diL_ref + RL*iL_ref + vc_ref*(1-u2) - x1*zeta1);
iL_ref_old = iL_ref;
vc_ref_old = vc_ref;

% compensate strategy
S1_duty_cycle = vc_ref / vin;
S4_duty_cycle = 1 - vin / vc_ref;  % vin < vc
S3_duty_cycle = 1- S4_duty_cycle;
PWM_triangular_wave_range = 2;
PWM_triangular_wave_min = -1;
original_u2 = u2;


persistent voltage_surge_max;
if isempty(voltage_surge_max)
    voltage_surge_max = 0;
end

if Bus_load > 1e2
    u2 = S4_duty_cycle;  % need to check
end


% Modify overshoot at initial stage
if vc - vc_ref > 1 %&& (vc - voltage_surge_max > -0.4)
    u2 = 2;
%     u2 = S3_duty_cycle * PWM_triangular_wave_range + PWM_triangular_wave_min;
    if vin - vc_ref > 1
        u1 = (1 - S1_duty_cycle) * PWM_triangular_wave_range + PWM_triangular_wave_min;
    end
end

% BoostMode
if vc_ref -vc > 0.5 % && Bus_load > 1e2
    u2 = S4_duty_cycle;
%     u2 = S3_duty_cycle * PWM_triangular_wave_range + PWM_triangular_wave_min;
    u1 = max(u1, S3_duty_cycle* PWM_triangular_wave_range + PWM_triangular_wave_min);
%     u1 = 2;
end


if abs(i_out) < 5 && abs(vc - vc_ref) < 0.3
    u2 = S4_duty_cycle;
end




% % Boost mode
% if (vc_ref - vin) > 1 && (vc_ref - vc) > 0.5
%     u1 = S1_duty_cycle * PWM_triangular_wave_range + PWM_triangular_wave_min;
% %     u2 = S4_duty_cycle * PWM_triangular_wave_range + PWM_triangular_wave_min;
% end
% 
% % Buck mode
% if vin - vc_ref > 1 && vc - vc_ref > 1
%     u2 = 2;
% %     u1 = S1_duty_cycle * PWM_triangular_wave_range + PWM_triangular_wave_min;
% end

voltage_surge_max = max(vc, voltage_surge_max);

== matlab function rectifire_single_inverter_pv1/battery/Battery and DC-DC converter/MATLAB Function1 ==
  settings: updateMethod=DISCRETE
  data: iL_ref input; u1 output; iL input; i_out_ref input; i_out input; vin input; Vc input; Ts input; u2 output
function [u1, u2] = Passivity_BC(iL_ref, iL,i_out_ref, i_out, vin, Vc, Ts)
% Constant output current Module
% param iL: inductor's current
% param iL_ref: expected value of inductor's current
% param i_out: dcdc output current 
% param i_out_ref
% param vin: input voltage
% param Vc: output voltage
%% system parameters
L = 40e-6;  % Inductance 电感 20uH
L_DMinductor = 2.2e-6;
L = L + L_DMinductor;
RL = 0.004;
C_output = 1440e-6;  % 电容大小

% zeta1 = 6*2;  % dumping gains
% zeta2 = 0.08*10;
zeta1 = L / RL * 2000;  % dumping gains
zeta2 = C_output * 1000; 

% error functions: state variable
x1 = iL - iL_ref;
x2 = i_out - i_out_ref;
persistent iL_ref_old Vc_old;
if isempty(iL_ref_old)
    iL_ref_old = 0;
    Vc_old = 0;
end

diL_ref = (iL_ref - iL_ref_old) / Ts;
dVc_ref = (Vc - Vc_old) / Ts;
%% calculate switching signal: u1,u2
u2 = 1 / iL_ref * (iL_ref - C_output * dVc_ref - i_out_ref + x2*zeta2);
u1 = 1 / vin * (L*diL_ref + RL * iL_ref + Vc * (1 - u2) - x1*zeta1);

iL_ref_old = iL_ref;
Vc_old = Vc;

== matlab function rectifire_single_inverter_pv1/battery/Battery and DC-DC converter/MATLAB Function2 ==
  settings: updateMethod=DISCRETE
  data: iL_ref input; u1 output; iL input; i_out_ref input; i_out input; vin input; Vc input; Ts input; u2 output
function [u1, u2] = Passivity_BC(iL_ref, iL,i_out_ref, i_out, vin, Vc, Ts)
% Constant output current Module
% param iL: inductor's current
% param iL_ref: expected value of inductor's current
% param i_out: dcdc output current 
% param i_out_ref
% param vin: input voltage
% param Vc: output voltage
%% system parameters
L = 40e-6;  % Inductance 电感 20uH
L_DMinductor = 2.2e-6;
L = L + L_DMinductor;
RL = 0.004;
C_output = 1440e-6;  % 电容大小

% zeta1 = 6 * 2;  % dumping gains
% zeta2 = 0.08 * 10;
zeta1 = L / RL * 2000;  % dumping gains
zeta2 = C_output * 1000; 

% error functions: state variable
x1 = iL - iL_ref;
x2 = i_out - i_out_ref;
persistent iL_ref_old Vc_old;
if isempty(iL_ref_old)
    iL_ref_old = 0;
    Vc_old = 0;
end

diL_ref = (iL_ref - iL_ref_old) / Ts;
dVc_ref = (Vc - Vc_old) / Ts;
%% calculate switching signal: u1,u2
u2 = 1 / iL_ref * (iL_ref - C_output * dVc_ref - i_out_ref + x2*zeta2);
u1 = 1 / vin * (L*diL_ref + RL * iL_ref + Vc * (1 - u2) - x1*zeta1);

iL_ref_old = iL_ref;
Vc_old = Vc;

== matlab function rectifire_single_inverter_pv1/battery/Battery and DC-DC converter/MATLAB Function3 ==
  settings: updateMethod=DISCRETE
  data: iL_ref input; u1 output; iL input; vc_ref input; vc input; vin input; i_out input; Ts input; u2 output
function [u1, u2] = Passivity_BC(iL_ref, iL, vc_ref, vc, vin, i_out, Ts)
% Constant output voltage Module
%   param vc_ref: expected
%   param vc: dcdc output voltage
%   param vin: input voltage
%   param io: current in output side
%% system parameters
L = 2 * 40e-6;  % Inductance 电感 20uH
L_DMinductor = 2.2e-6;
L = L + L_DMinductor;
RL = 0.004;
Co = 1440e-6;  % 电容大小

zeta1 = 6 * 2;  % dumping gains
zeta2 = 0.08 * 10; 

% error functions: state variable
x1 = iL - iL_ref;
x2 = vc - vc_ref;
persistent iL_ref_old vc_ref_old;
if isempty(iL_ref_old)
    iL_ref_old = 0;
    vc_ref_old = 0;
end

diL_ref = (iL_ref - iL_ref_old) / Ts;
dvc_ref = (vc_ref - vc_ref_old) / Ts;
%% calculate switching signal: u1,u2
u2 = 1 / iL_ref * (iL_ref - dvc_ref * Co - i_out + x2*zeta2);
u1 = 1 / vin * (L*diL_ref + RL*iL_ref + vc_ref*(1-u2) - x1*zeta1);
iL_ref_old = iL_ref;
vc_ref_old = vc_ref;

== matlab function rectifire_single_inverter_pv1/battery/Battery and DC-DC converter/MATLAB Function5 ==
  settings: updateMethod=DISCRETE
  data: iL_ref input; u1 output; iL input; i_out_ref input; i_out input; vin input; Vc input; Ts input; u2 output
function [u1, u2] = Passivity_BC(iL_ref, iL,i_out_ref, i_out, vin, Vc, Ts)
% Constant output current Module
% param iL: inductor's current
% param iL_ref: expected value of inductor's current
% param i_out: dcdc output current 
% param i_out_ref
% param vin: input voltage
% param Vc: output voltage
%% system parameters
L = 40e-6;  % Inductance 电感 20uH
L_DMinductor = 2.2e-6;
L = L + L_DMinductor;
RL = 0.004;
C_output = 1440e-6;  % 电容大小

zeta1 = 6;  % dumping gains
zeta2 = 0.08;

% error functions: state variable
x1 = iL - iL_ref;
x2 = i_out - i_out_ref;
persistent iL_ref_old Vc_old;
if isempty(iL_ref_old)
    iL_ref_old = 0;
    Vc_old = 0;
end

diL_ref = (iL_ref - iL_ref_old) / Ts;
dVc_ref = (Vc - Vc_old) / Ts;
%% calculate switching signal: u1,u2
u2 = 1 / iL_ref * (iL_ref - C_output * dVc_ref - i_out_ref + x2*zeta2);
u1 = 1 / vin * (L*diL_ref + RL * iL_ref + Vc * (1 - u2) - x1*zeta1);

iL_ref_old = iL_ref;
Vc_old = Vc;

== matlab function rectifire_single_inverter_pv1/battery/Battery and DC-DC converter/MATLAB Function6 ==
  settings: updateMethod=DISCRETE
  data: iL_ref input; u1 output; iL input; i_out_ref input; i_out input; vin input; Vc input; Ts input; u2 output
function [u1, u2] = Passivity_BC(iL_ref, iL,i_out_ref, i_out, vin, Vc, Ts)
% Constant output current Module
% param iL: inductor's current
% param iL_ref: expected value of inductor's current
% param i_out: dcdc output current 
% param i_out_ref
% param vin: input voltage
% param Vc: output voltage
%% system parameters
L = 40e-6;  % Inductance 电感 20uH
L_DMinductor = 2.2e-6;
L = L + L_DMinductor;
RL = 0.004;
C_output = 1440e-6;  % 电容大小

zeta1 = 6;  % dumping gains
zeta2 = 0.08;

% error functions: state variable
x1 = iL - iL_ref;
x2 = i_out - i_out_ref;
persistent iL_ref_old Vc_old;
if isempty(iL_ref_old)
    iL_ref_old = 0;
    Vc_old = 0;
end

diL_ref = (iL_ref - iL_ref_old) / Ts;
dVc_ref = (Vc - Vc_old) / Ts;
%% calculate switching signal: u1,u2
u2 = 1 / iL_ref * (iL_ref - C_output * dVc_ref - i_out_ref + x2*zeta2);
u1 = 1 / vin * (L*diL_ref + RL * iL_ref + Vc * (1 - u2) - x1*zeta1);

iL_ref_old = iL_ref;
Vc_old = Vc;
